simulink model "Thermal_model"  (R2021a)
settings: Solver=FixedStepAuto  StartTime=Qloss.time(1)  StopTime=Qloss.time(end)  FixedStep=1  RelTol=1e-3
undefined symbols (not defined in the file): Cth, CtoK, RealTemp, Rth
settings Model: Creator=keske  LastModifiedBy=cem
settings SolverCC: AlgebraicLoopSolver=TrustRegion
settings DebuggingCC: SFMachineParentedDataDiag=warning

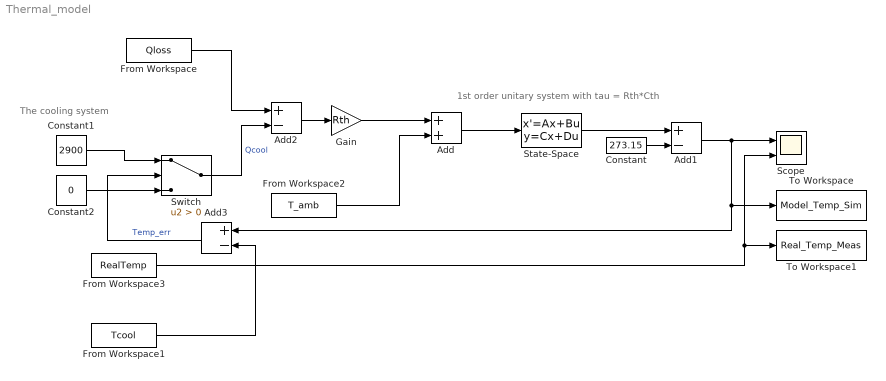
== system Thermal_model ==
  note: The cooling system
  note: 1st order unitary system with tau = Rth*Cth
  Add : Sum
  Add1 : Sum  Inputs=+-
  Add2 : Sum  Inputs=+-
  Add3 : Sum  Inputs=+-
  Constant : Constant  Value=273.15
  Constant1 : Constant  Value=2900
  Constant2 : Constant  Value=0
  From Workspace : FromWorkspace  VariableName=Qloss  SampleTime=1
  From Workspace1 : FromWorkspace  VariableName=Tcool  SampleTime=1
  From Workspace2 : FromWorkspace  VariableName=T_amb  SampleTime=1
  From Workspace3 : FromWorkspace  VariableName=RealTemp  SampleTime=1
  Gain : Gain  Gain=Rth
  Scope : Scope  NumInputPorts=2
  State-Space : StateSpace  A=-1/(Rth.*Cth)  B=1/(Rth.*Cth)  D=0  InitialCondition=RealTemp.Data(1) + CtoK
  Switch : Switch  Criteria=u2 > Threshold
  To Workspace : ToWorkspace  VariableName=Model_Temp_Sim  SaveFormat=Timeseries  SampleTime=-1
  To Workspace1 : ToWorkspace  VariableName=Real_Temp_Meas  SaveFormat=Timeseries  SampleTime=-1
  wires:
  From Workspace/1 -> Add2/1
  From Workspace2/1 -> Add/2
  Gain/1 -> Add/1
  Add1/1 -> Scope/1, To Workspace/1, Add3/1
  State-Space/1 -> Add1/1
  Add/1 -> State-Space/1
  Constant/1 -> Add1/2
  Add2/1 -> Gain/1
  From Workspace3/1 -> To Workspace1/1, Scope/2
  Constant1/1 -> Switch/1
  Constant2/1 -> Switch/3
  Switch/1 -> Add2/2  "Qcool"
  From Workspace1/1 -> Add3/2
  Add3/1 -> Switch/2  "Temp_err"
